simulink library "DTMFLibrary"  (R2019b)
settings: Solver=ode45  StartTime=0.0  StopTime=10.0  RelTol=1e-3  EnableMultiTasking=on
values from neighbouring files (symbols this model uses):
  dt = double(convertCharsToStrings(char(dt(1:end-1))))    [load_from_scope.m]
  Fs = 1/dt    [load_from_scope.m]
settings Model: Creator=Benn  LastModifiedBy=zceeash
settings DataIOCC: LimitDataPoints=on  SaveFormat=Array  ReturnWorkspaceOutputs=off
settings OptimizationCC: ExpressionDepthLimit=2147483647  LifeSpan=inf
settings DebuggingCC: UnderspecifiedInitializationDetection=Classic  MergeDetectMultiDrivingBlocksExec=none  SolverPrmCheckMsg=warning  MultiTaskDSMMsg=warning  MultiTaskCondExecSysMsg=none  FcnCallInpInsideContextMsg=warning  StateNameClashWarn=warning  SFUnexpectedBacktrackingDiag=warning  SFNoUnconditionalDefaultTransitionDiag=warning  SFExecutionAtInitializationDiag=none  ArithmeticOperatorsInVariantConditions=warning
settings HardwareCC: ProdBitPerPointer=32  ProdBitPerSizeT=32  ProdBitPerPtrDiffT=32  ProdLargestAtomicFloat=None  ProdIntDivRoundTo=Undefined  ProdEndianess=Unspecified  ProdWordSize=32  ProdHWDeviceType=32-bit Generic
settings ModelReferenceCC: PropagateSignalLabelsOutOfModel=off
settings SFSimCC: SimUseLocalCustomCode=off  CustomCodeUndefinedFunction=UseInterfaceOnly
settings RTWCC: RTWUseLocalCustomCode=off
settings CodeAppCC: StateflowObjectComments=on
settings GRTTargetCC: TargetLangStandard=C89/C90 (ANSI)  GeneratePreprocessorConditionals=Disable all
settings ConfigComp: CovMetricSettings=dw  CovHtmlReporting=on  CovSaveCumulativeToWorkspaceVar=on  CovSaveSingleToWorkspaceVar=on  CovExternalEMLEnable=off

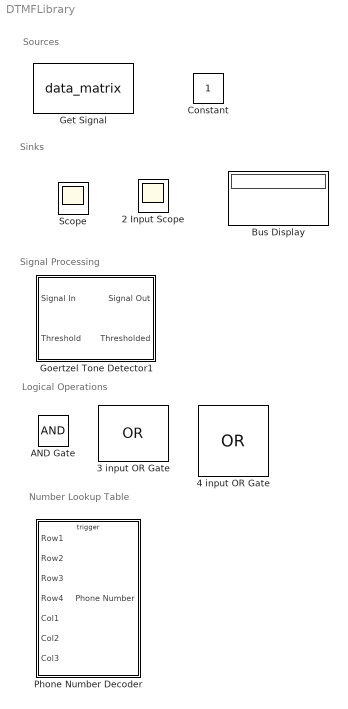
== system DTMFLibrary ==
  note: Sources
  note: Sinks
  note: Signal Processing
  note: Logical Operations
  note: Number Lookup Table
  2 Input Scope : Scope  NumInputPorts=2
  3 input OR Gate : Logic  Operator=OR  Inputs=3  AllPortsSameDT=off  OutDataTypeStr=boolean
  4 input OR Gate : Logic  Operator=OR  Inputs=4  AllPortsSameDT=off  OutDataTypeStr=boolean
  AND Gate : Logic  AllPortsSameDT=off  OutDataTypeStr=boolean
  Bus Display : Display
  Constant : Constant
  Get Signal : FromWorkspace  VariableName=data_matrix  SampleTime=dt  OutputAfterFinalValue=Setting to zero
      mask Display: disp('Oscilloscope Signal')
  Goertzel Tone Detector1 : Subsystem  AncestorBlock=UCAS/Goertzel Tone Detector  mask{ToneFreq=100, EstWindow=1}
      mask prompts: ToneFreq "Tone frequency (Hz)"; EstWindow "Estimation Window (s)"
      mask help: The sampling frequency Fs must be defined in the matlab command window e.g. Fs=8000;
      mask Display: disp(['Tone =' num2str(ToneFreq) ' Hz \n Time Window =' num2str(EstWindow)])
  Phone Number Decoder : Subsystem  TreatAsAtomicUnit=on
      mask help:
      | This block uses a lookup table to return the digit that is determined by the boolean state of the four row and three column inputs. Note only one of the row and column inputs can be true at any time.
      |
      | For example if row 2 and column 1 are both true then the digit 4 will be returned
  Scope : Scope

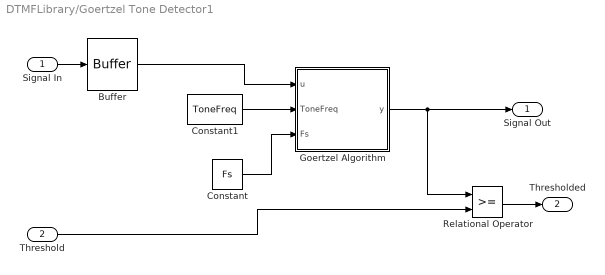
== system DTMFLibrary/Goertzel Tone Detector1 ==
  Signal In : Inport
  Threshold : Inport  Port=2
  Buffer : Buffer  N=ceil(EstWindow*Fs)
  Constant : Constant  Value=Fs
  Constant1 : Constant  Value=ToneFreq
  Goertzel Algorithm : MATLAB Function  TreatAsAtomicUnit=on
  Relational Operator : RelationalOperator  OutDataTypeStr=boolean  RndMeth=Nearest
  Signal Out : Outport
  Thresholded : Outport  Port=2
  wires:
  Relational Operator/1 -> Thresholded/1
  Threshold/1 -> Relational Operator/2
  Signal In/1 -> Buffer/1
  Buffer/1 -> Goertzel Algorithm/1(u)
  Goertzel Algorithm/1(y) -> Relational Operator/1, Signal Out/1
  Constant/1 -> Goertzel Algorithm/3(Fs)
  Constant1/1 -> Goertzel Algorithm/2(ToneFreq)

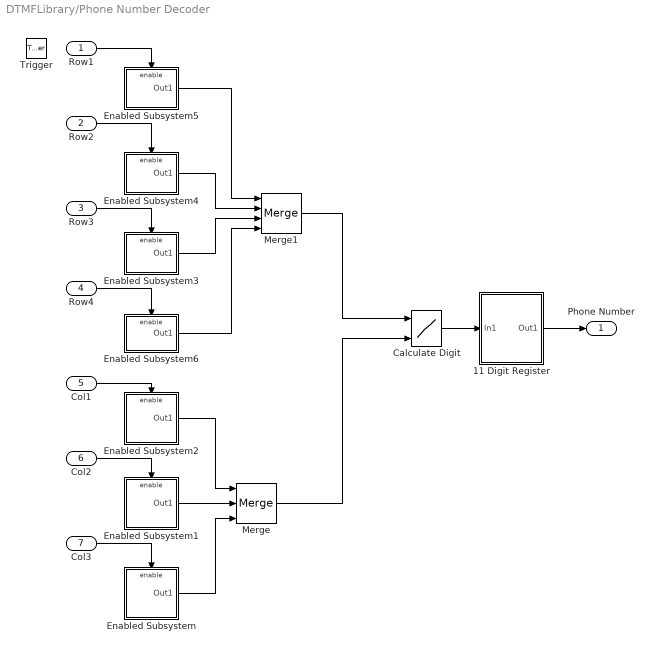
== system DTMFLibrary/Phone Number Decoder ==
  Row1 : Inport
  Row2 : Inport  Port=2
  Row3 : Inport  Port=3
  Row4 : Inport  Port=4
  Col1 : Inport  Port=5
  Col2 : Inport  Port=6
  Col3 : Inport  Port=7
  Trigger : TriggerPort  VariantControl=(inherit)
  11 Digit Register : Subsystem
  Calculate Digit : Lookup2D  RowIndex=[1:4]  ColumnIndex=[1:3]  Table=[1 2 3;4 5 6;7 8 9;10 0 11]  SaturateOnIntegerOverflow=on  InputSameDT=on
  Enabled Subsystem : Subsystem  TreatAsAtomicUnit=on
  Enabled Subsystem1 : Subsystem  TreatAsAtomicUnit=on
  Enabled Subsystem2 : Subsystem  TreatAsAtomicUnit=on
  Enabled Subsystem3 : Subsystem  TreatAsAtomicUnit=on
  Enabled Subsystem4 : Subsystem  TreatAsAtomicUnit=on
  Enabled Subsystem5 : Subsystem  TreatAsAtomicUnit=on
  Enabled Subsystem6 : Subsystem  TreatAsAtomicUnit=on
  Merge : Merge  Inputs=3
  Merge1 : Merge  Inputs=4
  Phone Number : Outport
  wires:
  Col3/1 -> Enabled Subsystem/Enable
  Col2/1 -> Enabled Subsystem1/Enable
  Col1/1 -> Enabled Subsystem2/Enable
  Enabled Subsystem2/1(Out1) -> Merge/1
  Enabled Subsystem1/1(Out1) -> Merge/2
  Enabled Subsystem/1(Out1) -> Merge/3
  Row3/1 -> Enabled Subsystem3/Enable
  Row2/1 -> Enabled Subsystem4/Enable
  Row1/1 -> Enabled Subsystem5/Enable
  Enabled Subsystem5/1(Out1) -> Merge1/1
  Enabled Subsystem4/1(Out1) -> Merge1/2
  Enabled Subsystem3/1(Out1) -> Merge1/3
  Row4/1 -> Enabled Subsystem6/Enable
  Enabled Subsystem6/1(Out1) -> Merge1/4
  Merge/1 -> Calculate Digit/2
  Merge1/1 -> Calculate Digit/1
  Calculate Digit/1 -> 11 Digit Register/1(In1)
  11 Digit Register/1(Out1) -> Phone Number/1

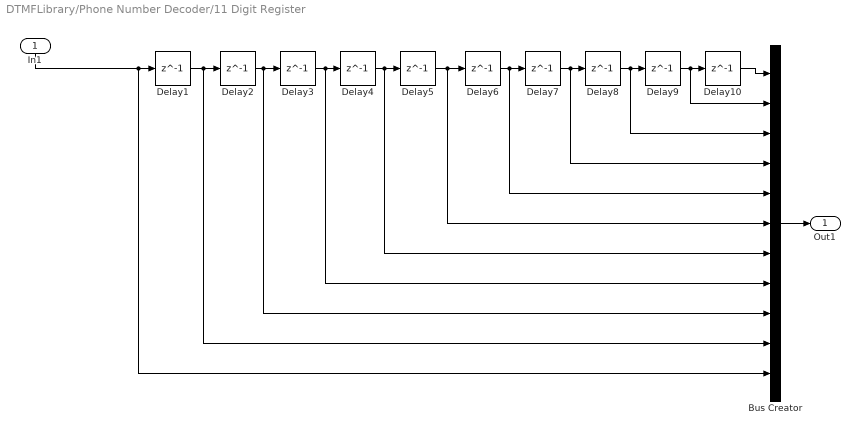
== system DTMFLibrary/Phone Number Decoder/11 Digit Register ==
  In1 : Inport
  Bus Creator : BusCreator  Inputs=11
  Delay{1..10} (10 alike) : Delay  DelayLength=1  InitialCondition=0
  Out1 : Outport
  wires:
  Delay9/1 -> Bus Creator/2, Delay10/1
  In1/1 -> Bus Creator/11, Delay1/1
  Delay2/1 -> Bus Creator/9, Delay3/1
  Delay8/1 -> Bus Creator/3, Delay9/1
  Delay4/1 -> Bus Creator/7, Delay5/1
  Delay3/1 -> Bus Creator/8, Delay4/1
  Delay6/1 -> Bus Creator/5, Delay7/1
  Delay5/1 -> Bus Creator/6, Delay6/1
  Delay7/1 -> Bus Creator/4, Delay8/1
  Delay1/1 -> Bus Creator/10, Delay2/1
  Delay10/1 -> Bus Creator/1
  Bus Creator/1 -> Out1/1

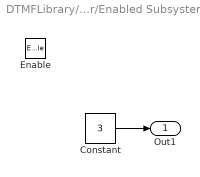
== system DTMFLibrary/Phone Number Decoder/Enabled Subsystem ==
  Enable : EnablePort
  Constant : Constant  Value=3
  Out1 : Outport
  wires:
  Constant/1 -> Out1/1

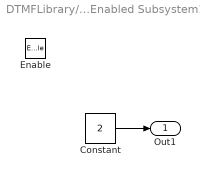
== system DTMFLibrary/Phone Number Decoder/Enabled Subsystem1 ==
  Enable : EnablePort
  Constant : Constant  Value=2
  Out1 : Outport
  wires:
  Constant/1 -> Out1/1

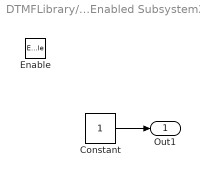
== system DTMFLibrary/Phone Number Decoder/Enabled Subsystem2 ==
  Enable : EnablePort
  Constant : Constant
  Out1 : Outport
  wires:
  Constant/1 -> Out1/1

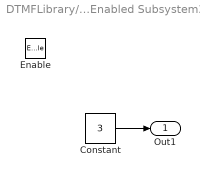
== system DTMFLibrary/Phone Number Decoder/Enabled Subsystem3 ==
  Enable : EnablePort
  Constant : Constant  Value=3
  Out1 : Outport
  wires:
  Constant/1 -> Out1/1

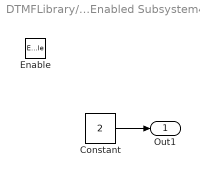
== system DTMFLibrary/Phone Number Decoder/Enabled Subsystem4 ==
  Enable : EnablePort
  Constant : Constant  Value=2
  Out1 : Outport
  wires:
  Constant/1 -> Out1/1

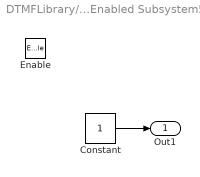
== system DTMFLibrary/Phone Number Decoder/Enabled Subsystem5 ==
  Enable : EnablePort
  Constant : Constant
  Out1 : Outport
  wires:
  Constant/1 -> Out1/1

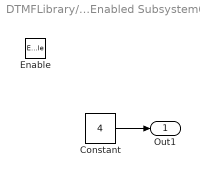
== system DTMFLibrary/Phone Number Decoder/Enabled Subsystem6 ==
  Enable : EnablePort
  Constant : Constant  Value=4
  Out1 : Outport
  wires:
  Constant/1 -> Out1/1

== matlab function DTMFLibrary/Goertzel Tone Detector1/Goertzel Algorithm ==
  data: u input; y output; ToneFreq input; Fs input
function y = fcn(u,ToneFreq,Fs)
%#codegen
N=length(u);
s1=0;
s2=0;
coeff=2*cos(2*pi*ToneFreq/Fs);
for n=1:N
    s=u(n)+coeff*s1-s2;
    s2=s1;
    s1=s;
end

y=(s2*s2+s1*s1-coeff*s1*s2)./N;
